simulink model "OR_10s_70l"  (R2023b)
settings: Solver=VariableStepAuto  StartTime=0.0  StopTime=10.0  RelTol=1e-3
undefined symbols (not defined in the file or in its folder): null
libraries: ABB_UPPAAL_Library x168
(part 3 of 3)

== matlab function OR_10s_70l/Bus_14 ==
  data: u input; y output
function y = fcn(u)

y = u;

== matlab function OR_10s_70l/Bus_1 ==
  data: u input; y output
function y = fcn(u)

y = u;

== matlab function OR_10s_70l/Bus_15 ==
  data: u input; y output
function y = fcn(u)

y = u;

== matlab function OR_10s_70l/Bus_16 ==
  data: u input; y output
function y = fcn(u)

y = u;

== matlab function OR_10s_70l/Bus_17 ==
  data: u input; y output
function y = fcn(u)

y = u;

== matlab function OR_10s_70l/Bus_18 ==
  data: u input; y output
function y = fcn(u)

y = u;

== matlab function OR_10s_70l/Bus_19 ==
  data: u input; y output
function y = fcn(u)

y = u;

== matlab function OR_10s_70l/Bus_20 ==
  data: u input; y output
function y = fcn(u)

y = u;

== matlab function OR_10s_70l/Bus_22 ==
  data: u input; y output
function y = fcn(u)

y = u;

== matlab function OR_10s_70l/Bus_23 ==
  data: data input; u input; y output
function y = fcn(data, u)

y = u;

== matlab function OR_10s_70l/Bus_24 ==
  data: data input; u input; y output
function y = fcn(data, u)

y = u;

== matlab function OR_10s_70l/Bus_21 ==
  data: data input; u input; y output
function y = fcn(data, u)

y = u;

== matlab function OR_10s_70l/Bus_2 ==
  data: u input; y output
function y = fcn(u)

y = u;

== matlab function OR_10s_70l/Bus_25 ==
  data: u input; y output
function y = fcn(u)

y = u;

== matlab function OR_10s_70l/Bus_26 ==
  data: u input; y output
function y = fcn(u)

y = u;

== matlab function OR_10s_70l/Bus_27 ==
  data: u input; y output
function y = fcn(u)

y = u;

== matlab function OR_10s_70l/Bus_28 ==
  data: u input; y output
function y = fcn(u)

y = u;

== matlab function OR_10s_70l/Bus_29 ==
  data: u input; y output
function y = fcn(u)

y = u;

== matlab function OR_10s_70l/Bus_30 ==
  data: u input; y output
function y = fcn(u)

y = u;

== matlab function OR_10s_70l/Bus_31 ==
  data: u input; y output
function y = fcn(u)

y = u;

== matlab function OR_10s_70l/Bus_32 ==
  data: data input; u input; y output
function y = fcn(data, u)

y = u;

== matlab function OR_10s_70l/Bus_33 ==
  data: u input; y output
function y = fcn(u)

y = u;

== matlab function OR_10s_70l/Bus_34 ==
  data: u input; y output
function y = fcn(u)

y = u;

== matlab function OR_10s_70l/Bus_3 ==
  data: u input; y output
function y = fcn(u)

y = u;

== matlab function OR_10s_70l/Bus_35 ==
  data: u input; y output
function y = fcn(u)

y = u;

== matlab function OR_10s_70l/Bus_36 ==
  data: u input; y output
function y = fcn(u)

y = u;

== matlab function OR_10s_70l/Bus_37 ==
  data: u input; y output
function y = fcn(u)

y = u;

== matlab function OR_10s_70l/Bus_38 ==
  data: u input; y output
function y = fcn(u)

y = u;

== matlab function OR_10s_70l/Bus_39 ==
  data: data input; u input; y output
function y = fcn(data, u)

y = u;

== matlab function OR_10s_70l/Bus_40 ==
  data: u input; y output
function y = fcn(u)

y = u;

== matlab function OR_10s_70l/Bus_41 ==
  data: u input; y output
function y = fcn(u)

y = u;

== matlab function OR_10s_70l/Bus_42 ==
  data: u input; y output
function y = fcn(u)

y = u;

== matlab function OR_10s_70l/Bus_43 ==
  data: u input; y output
function y = fcn(u)

y = u;

== matlab function OR_10s_70l/Bus_44 ==
  data: u input; y output
function y = fcn(u)

y = u;

== matlab function OR_10s_70l/Bus_4 ==
  data: data input; u input; y output
function y = fcn(data, u)

y = u;

== matlab function OR_10s_70l/Bus_45 ==
  data: u input; y output
function y = fcn(u)

y = u;

== matlab function OR_10s_70l/Bus_46 ==
  data: data input; u input; y output
function y = fcn(data, u)

y = u;

== matlab function OR_10s_70l/Bus_47 ==
  data: u input; y output
function y = fcn(u)

y = u;

== matlab function OR_10s_70l/Bus_48 ==
  data: u input; y output
function y = fcn(u)

y = u;

== matlab function OR_10s_70l/Bus_49 ==
  data: u input; y output
function y = fcn(u)

y = u;

== matlab function OR_10s_70l/Bus_50 ==
  data: u input; y output
function y = fcn(u)

y = u;

== matlab function OR_10s_70l/Bus_51 ==
  data: data input; u input; y output
function y = fcn(data, u)

y = u;

== matlab function OR_10s_70l/Bus_52 ==
  data: u input; y output
function y = fcn(u)

y = u;

== matlab function OR_10s_70l/Bus_53 ==
  data: u input; y output
function y = fcn(u)

y = u;

== matlab function OR_10s_70l/Bus_54 ==
  data: u input; y output
function y = fcn(u)

y = u;

== matlab function OR_10s_70l/Bus_55 ==
  data: u input; y output
function y = fcn(u)

y = u;

== matlab function OR_10s_70l/Bus_5 ==
  data: u input; y output
function y = fcn(u)

y = u;

== matlab function OR_10s_70l/Bus_56 ==
  data: u input; y output
function y = fcn(u)

y = u;

== matlab function OR_10s_70l/Bus_57 ==
  data: u input; y output
function y = fcn(u)

y = u;

== matlab function OR_10s_70l/Bus_58 ==
  data: u input; y output
function y = fcn(u)

y = u;

== matlab function OR_10s_70l/Bus_59 ==
  data: u input; y output
function y = fcn(u)

y = u;

== matlab function OR_10s_70l/Bus_60 ==
  data: u input; y output
function y = fcn(u)

y = u;

== matlab function OR_10s_70l/Bus_61 ==
  data: u input; y output
function y = fcn(u)

y = u;

== matlab function OR_10s_70l/Bus_62 ==
  data: u input; y output
function y = fcn(u)

y = u;

== matlab function OR_10s_70l/Bus_63 ==
  data: u input; y output
function y = fcn(u)

y = u;

== matlab function OR_10s_70l/Bus_64 ==
  data: u input; y output
function y = fcn(u)

y = u;

== matlab function OR_10s_70l/Bus_65 ==
  data: u input; y output
function y = fcn(u)

y = u;

== matlab function OR_10s_70l/Bus_6 ==
  data: u input; y output
function y = fcn(u)

y = u;

== matlab function OR_10s_70l/Bus_7 ==
  data: u input; y output
function y = fcn(u)

y = u;

== matlab function OR_10s_70l/Bus_8 ==
  data: u input; y output
function y = fcn(u)

y = u;

== matlab function OR_10s_70l/Bus_10 ==
  data: data input; u input; y output
function y = fcn(data, u)

y = u;

== matlab function OR_10s_70l/Bus_9 ==
  data: u input; y output
function y = fcn(u)

y = u;

== matlab function OR_10s_70l/Bus_11 ==
  data: u input; y output
function y = fcn(u)

y = u;

== matlab function OR_10s_70l/Bus_12 ==
  data: u input; y output
function y = fcn(u)

y = u;

== matlab function OR_10s_70l/Bus_13 ==
  data: u input; y output
function y = fcn(u)

y = u;
